simulink model "part2_MAIN_2019_working_EKF"  (R2023a)
settings: Solver=FixedStepAuto  StartTime=0.0  StopTime=500  FixedStep=0.1  RelTol=1e-3
values from neighbouring files (symbols this model uses):
  Af = diag(ti)    [init.m]    (also in init_old.m)
  change_position_time = 400    [init.m]    (also in init_old.m = 1200)
  Gamma = diag(omega_is)    [init.m]    (also in init_old.m)
  Kd = [1660451.40544401; 3920391.80535684; 1605063439.04156]    [init.m]    (also in init_old.m)
  Ki = [137.081306245593; 763.274947400198; 335358.448218978]    [init.m]    (also in init_old.m = [137.081306245593; 3163.274947400198; 335358.448218978])
  Kp = [75459.3345349083; 277551.73586971; 120744473.878042]    [init.m]    (also in init_old.m)
  Omega = diag([omega_n, omega_n, omega_n])    [get_observer_parameters.m]    (also in init.m = diag(2*omega_is.*zeta_is); init_old.m = diag(2*omega_is.*zeta_is))
  simulation = 1    [init.m]    (also in init_old.m)
  vessel =     [test.mat]
undefined symbols (not defined in the file or in its folder): Hoerner, thrusters
libraries: simulink x2, marine_hydro x2, marine_gnc x1
settings Model: PacingRate=8  Creator=jonbjor  LastModifiedBy=goks
settings SolverCC: AlgebraicLoopSolver=TrustRegion
settings DataIOCC: ReturnWorkspaceOutputs=off
settings DebuggingCC: AlgebraicLoopMsg=none  ArtificialAlgebraicLoopMsg=none  UnconnectedInputMsg=warning  UnconnectedOutputMsg=warning  UnconnectedLineMsg=warning  ArithmeticOperatorsInVariantConditions=warning
settings ModelReferenceCC: EnableRefExpFcnMdlSchedulingChecks=on
settings SFSimCC: SimUseLocalCustomCode=off  CustomCodeUndefinedFunction=UseInterfaceOnly
settings RTWCC: RTWUseLocalCustomCode=off  DLArmComputeVersion=19.05

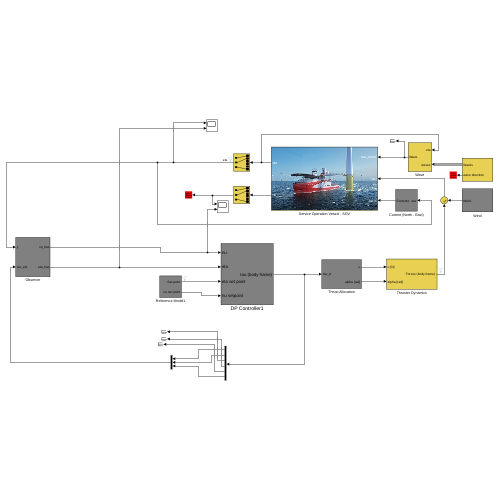
[thumbnail: Simulink's stored preview of the top-level diagram]
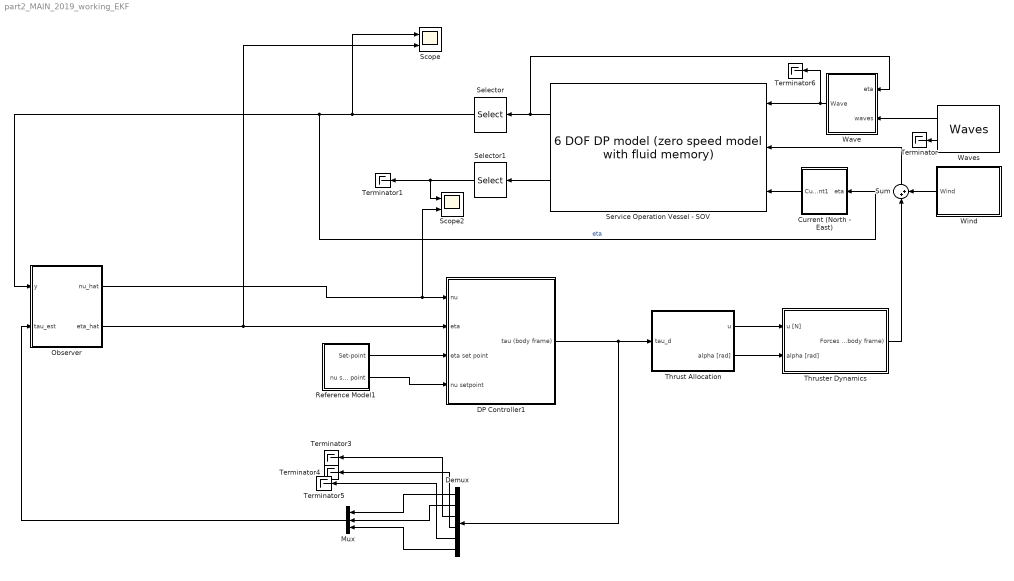
== system part2_MAIN_2019_working_EKF ==
  Current (North - East) : Subsystem
  DP Controller1 : Subsystem
  Demux : Demux  Outputs=6
  Mux : Mux  Inputs=3
  Observer : Subsystem
  Reference Model1 : Subsystem
  Scope : Scope  NumInputPorts=2
  Scope2 : Scope  NumInputPorts=2
  Selector : Selector  InputPortWidth=6  IndexOptions=Index vector (dialog)  Indices=[1 2 6]  OutputSizes=1
  Selector1 : Selector  InputPortWidth=6  IndexOptions=Index vector (dialog)  Indices=[1 2 6]  OutputSizes=1
  Service Operation Vessel - SOV : marine_hydro/Hydro Library/6 DOF DP model  (zero speed model with fluid memory)  ABC=vesselABC  rho=1025  Axc=0.9*vessel.main.T*vessel.main.B  Ayc=0.9*vessel.main.T*vessel.main.Lpp  CX=1  CY_2D=Hoerner(vessel.main.B,vessel.main.T)  Bv=vessel.Bv  mask(6 DOF zero speed model){}
      link override "Integrator1 ": InitialCondition=nu0
      link override Integrator2: InitialCondition=eta0
      mask Display:
      | image('SOV.jpg');
      | color('white'); port_label('output', 1, 'eta')
      | color('white'); port_label('output', 2, 'nu')
      | color('white'); port_label('input', 1, 'tau_wave')
      | color('white'); port_label('input', 2, 'tau')
      | color('white'); port_label('input', 3, 'nu_c')
  Sum : Sum  Inputs=|++
  Terminator{,1,3..6} (6 alike) : Terminator
  Thrust Allocation : Subsystem
  Thruster Dynamics : Subsystem  mask{thrusterfault=off}
      mask prompts: thrusterfault "Fault on thruster #2 and #4?"
  Wave : Subsystem  mask{waveforces=on}
      mask prompts: waveforces "Waveforces enabled"
  Waves : marine_gnc/Environment/Waves/Waves  spectrum_type=ITTC  disp_flag=on  plot_spectrum=off  plot_realization=off  hs=5  omega_peak=pi/10  psi_mean=0  gamma=-1  spread=2  depth=inf  nfreq=20  ndir=10  energylim=0.005  freq_cutoff=3  dir_cutoff=0  rand_seed=123  rand_freq=on  rand_dir=on  Zeta_a=0  Omega=0  Phase=0  Wavenum=0  Psi=0
  Wind : Subsystem
  wires:
  Service Operation Vessel - SOV/2 -> Selector1/1
  Reference Model1/1(Set-point) -> DP Controller1/3(eta set point)
  Service Operation Vessel - SOV/1 -> Wave/1(eta), Selector/1
  Waves/1 -> Wave/2(waves)
  Waves/2 -> Terminator/1
  Sum/1 -> Service Operation Vessel - SOV/2
  Selector/1 -> Scope/1, Current (North - East)/1(eta), Observer/1(y)  "eta"
  Reference Model1/2(nu set point) -> DP Controller1/4(nu setpoint)
  Selector1/1 -> Scope2/1, Terminator1/1
  Current (North - East)/1(Current1) -> Service Operation Vessel - SOV/3
  Wind/1(Wind) -> Sum/2
  Observer/1(nu_hat) -> Scope2/2, DP Controller1/1(nu)
  Demux/1 -> Mux/1
  Demux/2 -> Mux/2
  Demux/6 -> Mux/3
  Mux/1 -> Observer/2(tau_est)
  Demux/3 -> Terminator3/1
  Demux/4 -> Terminator4/1
  Demux/5 -> Terminator5/1
  Wave/1(Wave) -> Service Operation Vessel - SOV/1, Terminator6/1
  Observer/2(eta_hat) -> Scope/2, DP Controller1/2(eta)
  DP Controller1/1(tau (body frame)) -> Thrust Allocation/1(tau_d), Demux/1
  Thrust Allocation/1(u) -> Thruster Dynamics/1(u [N])
  Thruster Dynamics/1("Forces (body frame) ") -> Sum/1
  Thrust Allocation/2(alpha [rad]) -> Thruster Dynamics/2(alpha [rad])

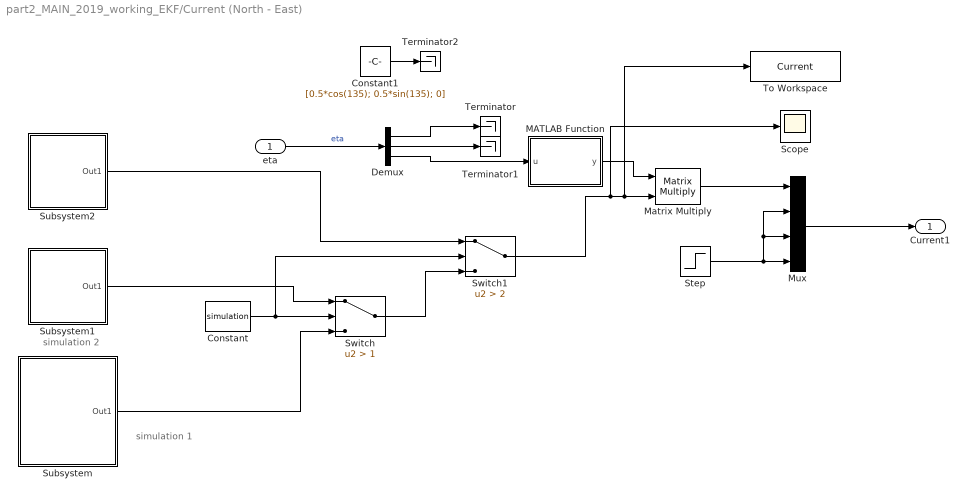
== system part2_MAIN_2019_working_EKF/Current (North - East) ==
  note: simulation 2
  note: simulation 1
  eta : Inport
  Constant : Constant  Value=simulation
  Constant1 : Constant  Value=[0.5*cos(135); 0.5*sin(135); 0]
  Demux : Demux  Outputs=3
  MATLAB Function : MATLAB Function  TreatAsAtomicUnit=on
  Matrix Multiply : Product  Multiplication=Matrix(*)
  Mux : Mux
  Scope : Scope
  Step : Step  After=0  SampleTime=0
  Subsystem : Subsystem
  Subsystem1 : Subsystem
  Subsystem2 : Subsystem
  Switch : Switch  Criteria=u2 > Threshold  Threshold=1  SaturateOnIntegerOverflow=off  InputSameDT=off
  Switch1 : Switch  Criteria=u2 > Threshold  Threshold=2  SaturateOnIntegerOverflow=off  InputSameDT=off
  Terminator : Terminator
  Terminator1 : Terminator
  Terminator2 : Terminator
  To Workspace : ToWorkspace  VariableName=Current  SaveFormat=Timeseries  SampleTime=-1
  Current1 : Outport  VectorParamsAs1DForOutWhenUnconnected=off
  wires:
  Demux/2 -> Terminator1/1
  MATLAB Function/1(y) -> Matrix Multiply/1
  Switch/1 -> Switch1/3
  Matrix Multiply/1 -> Mux/1
  Subsystem2/1(Out1) -> Switch1/1
  Subsystem/1(Out1) -> Switch/3
  Subsystem1/1(Out1) -> Switch/1
  Demux/1 -> Terminator/1
  Switch1/1 -> Scope/1, To Workspace/1, Matrix Multiply/2
  eta/1 -> Demux/1  "eta"
  Constant/1 -> Switch1/2, Switch/2
  Constant1/1 -> Terminator2/1
  Step/1 -> Mux/3, Mux/2, Mux/4
  Demux/3 -> MATLAB Function/1(u)
  Mux/1 -> Current1/1

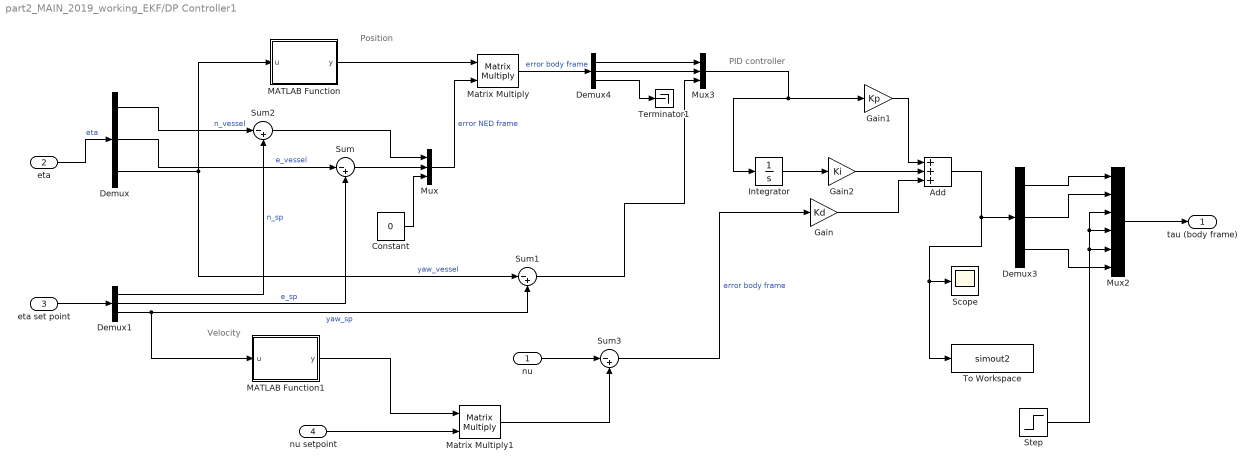
== system part2_MAIN_2019_working_EKF/DP Controller1 ==
  note: PID controller
  note: Velocity
  note: Position
  nu : Inport
  eta : Inport  Port=2
  eta set point : Inport  Port=3
  nu setpoint : Inport  Port=4
  Add : Sum  Inputs=+++
  Constant : Constant  Value=0
  Demux{,1,3..4} (4 alike) : Demux  Outputs=3
  Gain : Gain  Gain=Kd
  Gain1 : Gain  Gain=Kp
  Gain2 : Gain  Gain=Ki
  Integrator : Integrator
  MATLAB Function : MATLAB Function  TreatAsAtomicUnit=on
  MATLAB Function1 : MATLAB Function  TreatAsAtomicUnit=on
  Matrix Multiply : Product  Multiplication=Matrix(*)
  Matrix Multiply1 : Product  Multiplication=Matrix(*)
  Mux : Mux  Inputs=3
  Mux2 : Mux  Inputs=6
  Mux3 : Mux  Inputs=3
  Scope : Scope
  Step : Step  After=0  SampleTime=0
  Sum{,1..3} (4 alike) : Sum  Inputs=|-+
  Terminator1 : Terminator
  To Workspace : ToWorkspace  VariableName=simout2  SaveFormat=Timeseries  SampleTime=-1
  tau (body frame) : Outport  VectorParamsAs1DForOutWhenUnconnected=off
  wires:
  eta/1 -> Demux/1  "eta"
  eta set point/1 -> Demux1/1
  Demux/1 -> Sum2/1  "n_vessel"
  Demux1/1 -> Sum2/2  "n_sp"
  Demux/2 -> Sum/1  "e_vessel"
  Demux1/2 -> Sum/2  "e_sp"
  Sum2/1 -> Mux/1
  Sum/1 -> Mux/2
  MATLAB Function/1(y) -> Matrix Multiply/1
  Mux/1 -> Matrix Multiply/2  "error NED frame"
  Step/1 -> Mux2/4, Mux2/3, Mux2/5
  Demux1/3 -> MATLAB Function1/1(u), Sum1/2  "yaw_sp"
  Sum1/1 -> Mux3/3
  Constant/1 -> Mux/3
  Demux/3 -> Sum1/1, MATLAB Function/1(u)  "yaw_vessel"
  Matrix Multiply/1 -> Demux4/1  "error body frame"
  nu/1 -> Sum3/1
  Sum3/1 -> Gain/1  "error body frame"
  nu setpoint/1 -> Matrix Multiply1/2
  MATLAB Function1/1(y) -> Matrix Multiply1/1
  Matrix Multiply1/1 -> Sum3/2
  Integrator/1 -> Gain2/1
  Gain1/1 -> Add/1
  Gain2/1 -> Add/2
  Gain/1 -> Add/3
  Add/1 -> To Workspace/1, Scope/1, Demux3/1
  Demux3/1 -> Mux2/1
  Demux3/2 -> Mux2/2
  Demux3/3 -> Mux2/6
  Mux2/1 -> tau (body frame)/1
  Demux4/1 -> Mux3/1
  Demux4/2 -> Mux3/2
  Demux4/3 -> Terminator1/1
  Mux3/1 -> Integrator/1, Gain1/1

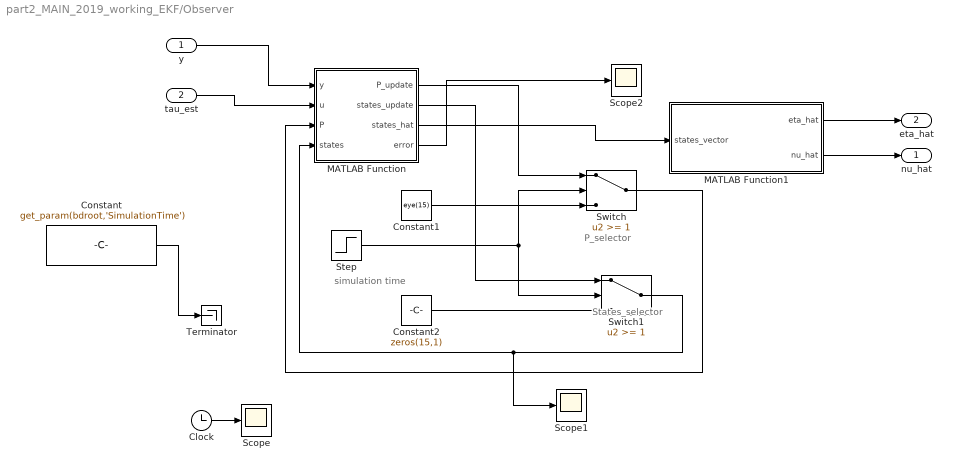
== system part2_MAIN_2019_working_EKF/Observer ==
  note: simulation time
  note: States_selector
  note: P_selector
  y : Inport
  tau_est : Inport  Port=2
  Clock : Clock
  Constant : Constant  Value=get_param(bdroot,'SimulationTime')
  Constant1 : Constant  Value=eye(15)
  Constant2 : Constant  Value=zeros(15,1)
  MATLAB Function : MATLAB Function  TreatAsAtomicUnit=on
  MATLAB Function1 : MATLAB Function  TreatAsAtomicUnit=on
  Scope : Scope
  Scope1 : Scope
  Scope2 : Scope
  Step : Step  Time=0.01  SampleTime=0.1
  Switch : Switch  Threshold=1  SaturateOnIntegerOverflow=off  InputSameDT=off
  Switch1 : Switch  Threshold=1  SaturateOnIntegerOverflow=off  InputSameDT=off
  Terminator : Terminator
  nu_hat : Outport  VectorParamsAs1DForOutWhenUnconnected=off
  eta_hat : Outport  Port=2  VectorParamsAs1DForOutWhenUnconnected=off
  wires:
  tau_est/1 -> MATLAB Function/2(u)
  MATLAB Function/1(P_update) -> Switch/1
  Constant1/1 -> Switch/3
  Constant2/1 -> Switch1/3
  MATLAB Function/2(states_update) -> Switch1/1
  y/1 -> MATLAB Function/1(y)
  Switch/1 -> MATLAB Function/3(P)
  Switch1/1 -> Scope1/1, MATLAB Function/4(states)
  MATLAB Function1/1(eta_hat) -> eta_hat/1
  MATLAB Function1/2(nu_hat) -> nu_hat/1
  Step/1 -> Switch1/2, Switch/2
  Constant/1 -> Terminator/1
  Clock/1 -> Scope/1
  MATLAB Function/3(states_hat) -> MATLAB Function1/1(states_vector)
  MATLAB Function/4(error) -> Scope2/1

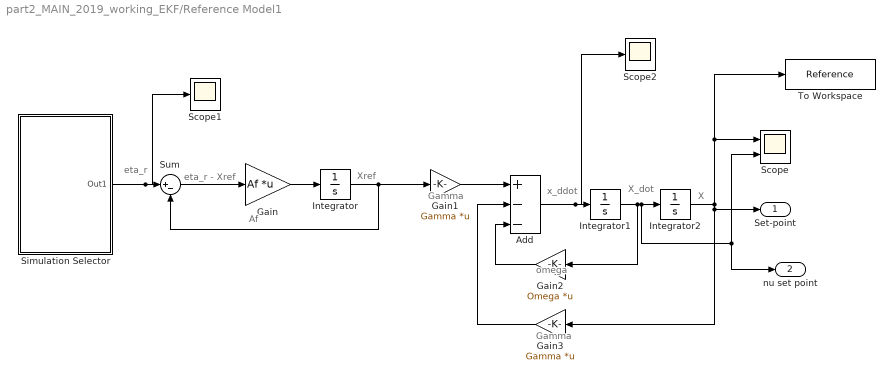
== system part2_MAIN_2019_working_EKF/Reference Model1 ==
  note: Af
  note: eta_r
  note: Xref
  note: omega
  note: eta_r - Xref
  note: Gamma
  note: x_ddot
  note: Gamma
  note: X_dot
  note: X
  Add : Sum  Inputs=+--
  Gain : Gain  Gain=Af  Multiplication=Matrix(K*u)
  Gain1 : Gain  Gain=Gamma  Multiplication=Matrix(K*u)
  Gain2 : Gain  Gain=Omega  Multiplication=Matrix(K*u)
  Gain3 : Gain  Gain=Gamma  Multiplication=Matrix(K*u)
  Integrator : Integrator
  Integrator1 : Integrator
  Integrator2 : Integrator
  Scope : Scope  NumInputPorts=2
  Scope1 : Scope
  Scope2 : Scope
  Simulation Selector : Subsystem
  Sum : Sum  Inputs=|+-
  To Workspace : ToWorkspace  VariableName=Reference  SaveFormat=Timeseries  SampleTime=-1
  Set-point : Outport  VectorParamsAs1DForOutWhenUnconnected=off
  nu set point : Outport  Port=2  VectorParamsAs1DForOutWhenUnconnected=off
  wires:
  Integrator/1 -> Gain1/1, Sum/2
  Add/1 -> Scope2/1, Integrator1/1
  Integrator2/1 -> To Workspace/1, Scope/1, Set-point/1, Gain3/1
  Gain1/1 -> Add/1
  Integrator1/1 -> nu set point/1, Scope/2, Integrator2/1, Gain2/1
  Gain/1 -> Integrator/1
  Gain2/1 -> Add/3
  Gain3/1 -> Add/2
  Simulation Selector/1(Out1) -> Scope1/1, Sum/1
  Sum/1 -> Gain/1

== system part2_MAIN_2019_working_EKF/Thrust Allocation ==
  tau_d : Inport
  MATLAB Function : MATLAB Function  TreatAsAtomicUnit=on
  u : Outport  VectorParamsAs1DForOutWhenUnconnected=off
  alpha [rad] : Outport  Port=2  VectorParamsAs1DForOutWhenUnconnected=off
  wires:
  tau_d/1 -> MATLAB Function/1(tau_d)
  MATLAB Function/1(Td) -> u/1
  MATLAB Function/2(alpha) -> alpha [rad]/1

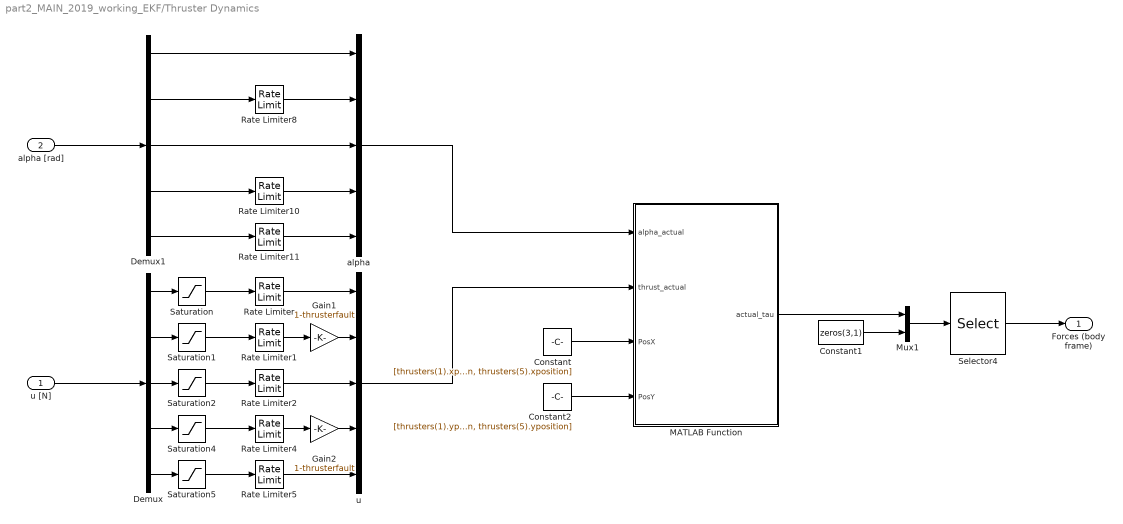
== system part2_MAIN_2019_working_EKF/Thruster Dynamics ==
  u [N] : Inport
  alpha [rad] : Inport  Port=2
  Constant : Constant  Value=[thrusters(1).xposition, thrusters(2).xposition, thrusters(3).xposition, thrusters(4).xposition, thrusters(5).xposition]
  Constant1 : Constant  Value=zeros(3,1)
  Constant2 : Constant  Value=[thrusters(1).yposition, thrusters(2).yposition, thrusters(3).yposition, thrusters(4).yposition, thrusters(5).yposition]
  Demux : Demux  Outputs=5
  Demux1 : Demux  Outputs=5
  Gain1 : Gain  Gain=1-thrusterfault
  Gain2 : Gain  Gain=1-thrusterfault
  MATLAB Function : MATLAB Function  TreatAsAtomicUnit=on
  Mux1 : Mux  Inputs=2
  Rate Limiter : RateLimiter  RisingSlewLimit=thrusters(1).rate  FallingSlewLimit=-thrusters(1).rate  SampleTimeMode=inherited
  Rate Limiter1 : RateLimiter  RisingSlewLimit=thrusters(2).rate  FallingSlewLimit=-thrusters(2).rate  SampleTimeMode=inherited
  Rate Limiter10 : RateLimiter  RisingSlewLimit=thrusters(4).rotationspeed  FallingSlewLimit=-thrusters(4).rotationspeed  SampleTimeMode=inherited
  Rate Limiter11 : RateLimiter  RisingSlewLimit=thrusters(5).rotationspeed  FallingSlewLimit=-thrusters(5).rotationspeed  SampleTimeMode=inherited
  Rate Limiter2 : RateLimiter  RisingSlewLimit=thrusters(3).rate  FallingSlewLimit=-thrusters(3).rate  SampleTimeMode=inherited
  Rate Limiter4 : RateLimiter  RisingSlewLimit=thrusters(4).rate  FallingSlewLimit=-thrusters(4).rate  SampleTimeMode=inherited
  Rate Limiter5 : RateLimiter  RisingSlewLimit=thrusters(5).rate  FallingSlewLimit=-thrusters(5).rate  SampleTimeMode=inherited
  Rate Limiter8 : RateLimiter  RisingSlewLimit=thrusters(2).rotationspeed  FallingSlewLimit=-thrusters(2).rotationspeed  SampleTimeMode=inherited
  Saturation : Saturate  UpperLimit=thrusters(1).thrust  LowerLimit=-thrusters(1).thrust
  Saturation1 : Saturate  UpperLimit=thrusters(2).thrust  LowerLimit=-thrusters(2).thrust
  Saturation2 : Saturate  UpperLimit=thrusters(3).thrust  LowerLimit=-thrusters(3).thrust
  Saturation4 : Saturate  UpperLimit=thrusters(4).thrust  LowerLimit=-thrusters(4).thrust
  Saturation5 : Saturate  UpperLimit=thrusters(5).thrust  LowerLimit=-thrusters(5).thrust
  Selector4 : Selector  InputPortWidth=6  IndexOptions=Index vector (dialog)  Indices=[1 2 4 5 6 3]  OutputSizes=1
  alpha : Mux  Inputs=5
  u : Mux  Inputs=5
  "Forces (body frame) " : Outport  VectorParamsAs1DForOutWhenUnconnected=off
  wires:
  Rate Limiter2/1 -> u/3
  Saturation/1 -> Rate Limiter/1
  Mux1/1 -> Selector4/1
  Constant1/1 -> Mux1/2
  Saturation4/1 -> Rate Limiter4/1
  Demux/2 -> Saturation1/1
  Saturation1/1 -> Rate Limiter1/1
  Demux/1 -> Saturation/1
  Demux/3 -> Saturation2/1
  Saturation2/1 -> Rate Limiter2/1
  Selector4/1 -> "Forces (body frame) "/1
  Gain1/1 -> u/2
  Rate Limiter1/1 -> Gain1/1
  Rate Limiter/1 -> u/1
  Rate Limiter4/1 -> Gain2/1
  Saturation5/1 -> Rate Limiter5/1
  u [N]/1 -> Demux/1
  alpha [rad]/1 -> Demux1/1
  Constant/1 -> MATLAB Function/3(PosX)
  Constant2/1 -> MATLAB Function/4(PosY)
  u/1 -> MATLAB Function/2(thrust_actual)
  alpha/1 -> MATLAB Function/1(alpha_actual)
  MATLAB Function/1(actual_tau) -> Mux1/1
  Rate Limiter10/1 -> alpha/4
  Demux1/4 -> Rate Limiter10/1
  Demux1/5 -> Rate Limiter11/1
  Rate Limiter11/1 -> alpha/5
  Demux1/1 -> alpha/1
  Gain2/1 -> u/4
  Demux/4 -> Saturation4/1
  Demux/5 -> Saturation5/1
  Rate Limiter5/1 -> u/5
  Demux1/2 -> Rate Limiter8/1
  Rate Limiter8/1 -> alpha/2
  Demux1/3 -> alpha/3

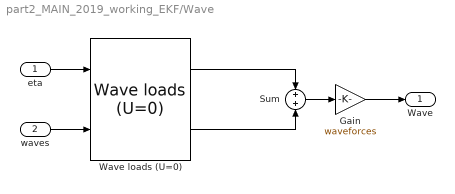
== system part2_MAIN_2019_working_EKF/Wave ==
  eta : Inport
  waves : Inport  Port=2
  Gain : Gain  Gain=waveforces
  Sum : Sum
  Wave loads (U=0) : marine_hydro/Hydro Library/Wave loads (U=0)  SystemSampleTime=-1  VariantActivationTime=update diagram  Latency=0  AutoFrameSizeCalculation=off
  Wave : Outport  VectorParamsAs1DForOutWhenUnconnected=off
  wires:
  eta/1 -> Wave loads (U=0)/1
  waves/1 -> Wave loads (U=0)/2
  Sum/1 -> Gain/1
  Wave loads (U=0)/1 -> Sum/1
  Wave loads (U=0)/2 -> Sum/2
  Gain/1 -> Wave/1

== system part2_MAIN_2019_working_EKF/Wind ==
  Constant : Constant  Value=zeros(6,1)
  Wind : Outport  VectorParamsAs1DForOutWhenUnconnected=off
  wires:
  Constant/1 -> Wind/1

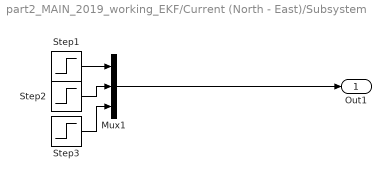
== system part2_MAIN_2019_working_EKF/Current (North - East)/Subsystem ==
  Mux1 : Mux  Inputs=3
  Step1 : Step  Time=0  After=0.5*cos(135)  SampleTime=0
  Step2 : Step  Time=0  After=0.5*sin(135)  SampleTime=0
  Step3 : Step  Time=0  After=0  SampleTime=0
  Out1 : Outport
  wires:
  Mux1/1 -> Out1/1
  Step1/1 -> Mux1/1
  Step2/1 -> Mux1/2
  Step3/1 -> Mux1/3

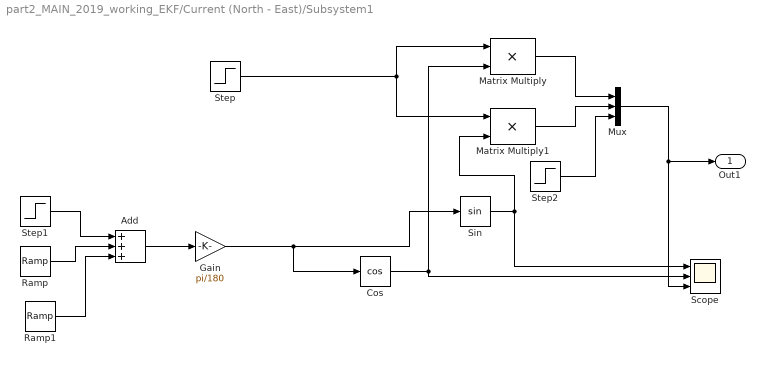
== system part2_MAIN_2019_working_EKF/Current (North - East)/Subsystem1 ==
  Add : Sum  Inputs=+++
  Cos : Trigonometry  Operator=cos
  Gain : Gain  Gain=pi/180
  Matrix Multiply : Product
  Matrix Multiply1 : Product
  Mux : Mux  Inputs=3
  Ramp : simulink/Sources/Ramp  slope=0.45  start=2  InitialOutput=0
  Ramp1 : simulink/Sources/Ramp  slope=-0.45  start=202  InitialOutput=0
  Scope : Scope  NumInputPorts=3
  Sin : Trigonometry
  Step : Step  Time=2  After=0.5  SampleTime=0
  Step1 : Step  Time=2  Before=180  After=180  SampleTime=0
  Step2 : Step  Time=0  After=0  SampleTime=0
  Out1 : Outport
  wires:
  Step1/1 -> Add/1
  Ramp/1 -> Add/2
  Ramp1/1 -> Add/3
  Step/1 -> Matrix Multiply1/1, Matrix Multiply/1
  Sin/1 -> Matrix Multiply1/2, Scope/1
  Cos/1 -> Matrix Multiply/2, Scope/2
  Matrix Multiply/1 -> Mux/1
  Matrix Multiply1/1 -> Mux/2
  Step2/1 -> Mux/3
  Mux/1 -> Scope/3, Out1/1
  Add/1 -> Gain/1
  Gain/1 -> Sin/1, Cos/1

== system part2_MAIN_2019_working_EKF/Current (North - East)/Subsystem2 ==
  Mux : Mux  Inputs=3
  Step : Step  Time=0  After=0  SampleTime=0
  Out1 : Outport
  wires:
  Mux/1 -> Out1/1
  Step/1 -> Mux/3, Mux/2, Mux/1

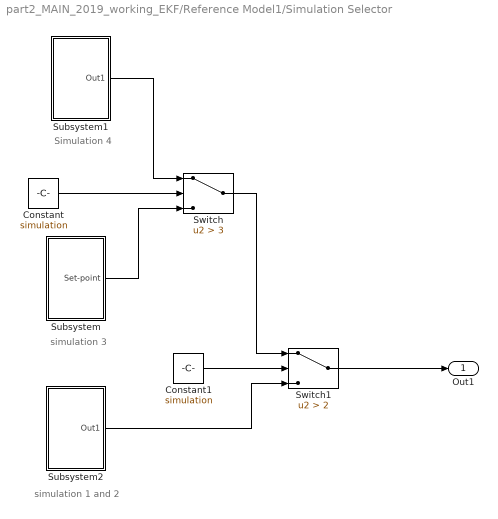
== system part2_MAIN_2019_working_EKF/Reference Model1/Simulation Selector ==
  note: simulation 1 and 2
  note: Simulation 4
  note: simulation 3
  Constant : Constant  Value=simulation
  Constant1 : Constant  Value=simulation
  Subsystem : Subsystem
  Subsystem1 : Subsystem
  Subsystem2 : Subsystem
  Switch : Switch  Criteria=u2 > Threshold  Threshold=3  SaturateOnIntegerOverflow=off  InputSameDT=off
  Switch1 : Switch  Criteria=u2 > Threshold  Threshold=2  SaturateOnIntegerOverflow=off  InputSameDT=off
  Out1 : Outport
  wires:
  Subsystem1/1(Out1) -> Switch/1
  Subsystem/1(Set-point) -> Switch/3
  Constant/1 -> Switch/2
  Switch/1 -> Switch1/1
  Constant1/1 -> Switch1/2
  Subsystem2/1(Out1) -> Switch1/3
  Switch1/1 -> Out1/1

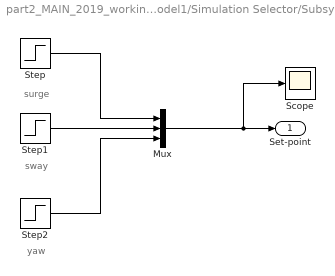
== system part2_MAIN_2019_working_EKF/Reference Model1/Simulation Selector/Subsystem ==
  note: yaw
  note: sway
  note: surge
  Mux : Mux  Inputs=3
  Scope : Scope
  Step : Step  After=10  SampleTime=0
  Step1 : Step  After=10  SampleTime=0
  Step2 : Step  After=3*pi/2  SampleTime=0
  Set-point : Outport
  wires:
  Step/1 -> Mux/1
  Step1/1 -> Mux/2
  Step2/1 -> Mux/3
  Mux/1 -> Scope/1, Set-point/1

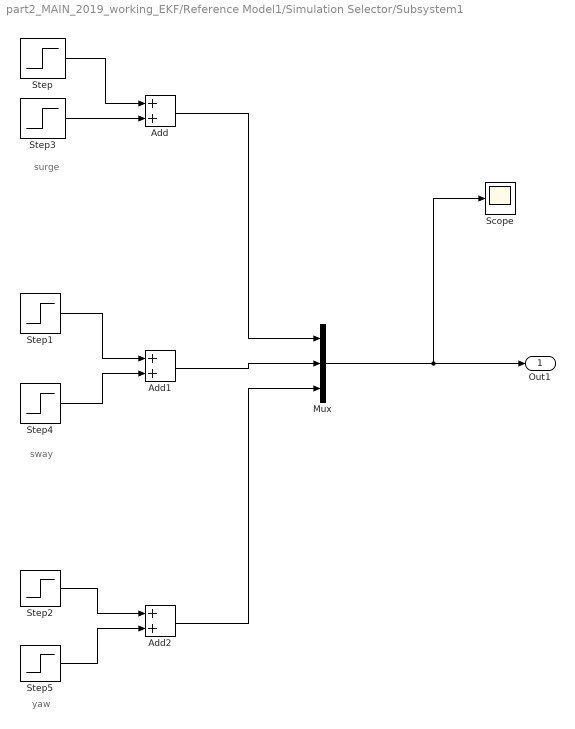
== system part2_MAIN_2019_working_EKF/Reference Model1/Simulation Selector/Subsystem1 ==
  note: yaw
  note: sway
  note: surge
  Add : Sum
  Add1 : Sum
  Add2 : Sum
  Mux : Mux  Inputs=3
  Scope : Scope
  Step : Step  Time=10  After=50  SampleTime=0
  Step1 : Step  Time=change_position_time  After=-50  SampleTime=0
  Step2 : Step  Time=change_position_time*2  After=pi/4  SampleTime=0
  Step3 : Step  Time=change_position_time*3  After=-50  SampleTime=0
  Step4 : Step  Time=change_position_time*4  After=50  SampleTime=0
  Step5 : Step  Time=change_position_time*4  After=-pi/4  SampleTime=0
  Out1 : Outport
  wires:
  Mux/1 -> Scope/1, Out1/1
  Step/1 -> Add/1
  Step3/1 -> Add/2
  Step1/1 -> Add1/1
  Step4/1 -> Add1/2
  Step2/1 -> Add2/1
  Step5/1 -> Add2/2
  Add/1 -> Mux/1
  Add1/1 -> Mux/2
  Add2/1 -> Mux/3

== system part2_MAIN_2019_working_EKF/Reference Model1/Simulation Selector/Subsystem2 ==
  Mux : Mux  Inputs=3
  Step : Step  After=0  SampleTime=0
  Step1 : Step  After=0  SampleTime=0
  Step2 : Step  After=0  SampleTime=0
  Out1 : Outport
  wires:
  Step/1 -> Mux/1
  Step1/1 -> Mux/2
  Step2/1 -> Mux/3
  Mux/1 -> Out1/1

== matlab function part2_MAIN_2019_working_EKF/Current (North - East)/MATLAB Function ==
  data: u input; y output
function y = fcn(u)
rot = [cos(u) -sin(u) 0;
    sin(u) cos(u) 0;
    0 0 1];

y = rot';

== matlab function part2_MAIN_2019_working_EKF/DP Controller1/MATLAB Function ==
  data: u input; y output
function y = fcn(u)

rot = [cos(u) -sin(u) 0;
    sin(u) cos(u) 0;
    0 0 1];

y = rot';

== matlab function part2_MAIN_2019_working_EKF/DP Controller1/MATLAB Function1 ==
  data: u input; y output
function y = fcn(u)

rot = [cos(u) -sin(u) 0;
    sin(u) cos(u) 0;
    0 0 1];

y = rot';

== matlab function part2_MAIN_2019_working_EKF/Observer/MATLAB Function1 ==
  data: states_vector input; eta_hat output; nu_hat output
function [eta_hat, nu_hat] = fcn(states_vector)
%%states [zeta,eta, b, nu] --15x1
%zeta - 6x1, 
%eta - 3x1, 
%b - 3x1, 
%nu - 3x1
eta_hat = states_vector(7:9,1);
nu_hat = states_vector(13:15,1);

end

== matlab function part2_MAIN_2019_working_EKF/Observer/MATLAB Function ==
  data: y input; u input; P input; P_update output; states input; states_update output; states_hat output; error output
function [P_update, states_update,states_hat,error]= fcn(y, u, P, states)
%%%P - 15x15
%states [zeta,eta, b, nu] --15x1
%zeta - 6x1, 
%eta - 3x1, 
%b - 3x1, 
%nu - 3x1
%u - 3x1 force input 
%
%ws_var containing other matrices
%Aw, Tb, B, E, H

%%%all the variables
T_n = 20; %period of interest -- can tune
omega_n = 2* pi / T_n;
zeta = 0.1; %--- can tune
Omega = diag([omega_n, omega_n, omega_n]);
Caret = diag([zeta, zeta, zeta]);
Tb = 0.1 * eye(3); %tune the 0.1
A_w =  [zeros(3) eye(3);
    -Omega^2 -2*Caret*Omega];

ws_var.Aw = A_w;


C_w = [zeros(3) eye(3)];
ws_var.Cw = C_w;



K_w = diag([1, 1, 1]); %-------TUNE
E_w = [zeros(3); K_w];
ws_var.Ew = E_w;
E_b = diag([1, 1, 1]); %-----TUNE 
% Mass = diag([vesselABC.MRB(1,1), vesselABC.MRB(2,2), vesselABC.MRB(6,6)]); %vesselABC.MRB(1:3,1:3);

ws_var.Eb = E_b;
Mass =    [7.0101e+06  0            0;
            0    8.519e+06   4.7187e+05;
            0  4.7187e+05   3.7973e+09];
Damping = diag([2.6486e5, 8.8164e5, 3.3774e8]);
ws_var.M = Mass;
ws_var.D = Damping;

ws_var.B =  [zeros(6,3);zeros(3,3);zeros(3,3);inv(Mass)];
ws_var.E = [E_w, zeros(6,3);
            zeros(3,3), zeros(3,3);
            zeros(3,3), E_b;
            zeros(3,3),zeros(3,3)];
ws_var.H = [C_w, eye(3), zeros(3,3) zeros(3,3)];
ws_var.Tb = Tb;
ws_var.init_state = zeros(15,1);
ws_var.init_Pk = 0.1*eye(15); %tune later
ws_var.R = diag([1,1,0.1]); %tune later
ws_var.Q = diag([1,1,0.1,1e4,1e4,1e5]); %tune this
ws_var.dt = 0.1; %get from simulink fixed step

%%%

H =ws_var.H;
R = ws_var.R;
% y = states(7:9,1);
%predictor
phi = PHI(states,ws_var.dt, ws_var);
TAU = ws_var.dt*ws_var.E;
P_hat = phi*P*phi' + TAU*ws_var.Q*TAU';
states_hat = states+ws_var.dt*F_x_u(states,u, ws_var);


%corrector
%kalman gain
K = P_hat*H'*inv(H*P_hat*H'+R);
P_update = (eye(15)-K*H)*P_hat*(eye(15)-K*H)' + K*R*K';
states_update = states_hat + K*(y-H*states_hat);
error = y - H*states_hat;
end



function phis = PHI(states,dt,ws_var)
%%%states [zeta,eta, b, nu] --15x1
%zeta - 6x1, 
%eta - 3x1, 
%b - 3x1, 
%nu - 3x1
%%%u - 3x1 force input
%%%D - damping, M - Mass, 
%ws_var containing other matrices
%Aw, Tb, B, E, H
zeta = states(1:6,:);
eta = states(7:9,:);
b = states(10:12,:);
nu = states(13:15,:);

psi = eta(3,1);
Jrot = zeros(3,3);
Jrot(1,3) = -cos(psi)*nu(2,1)-sin(psi)*nu(1,1);
Jrot(2,3) = cos(psi)*nu(1,1) - sin(psi)*nu(2,1);

R = [cos(eta(3,1)) -sin(eta(3,1)) 0;
    sin(eta(3,1)) cos(eta(3,1)) 0;
    0 0 1];

phi = zeros(15,15);
phi(1:6,1:6) = ws_var.Aw;
phi(7:9, 7:9) = Jrot;
phi(7:9, 13:15) = R;

phi(10:12, 10:12) = -inv(ws_var.Tb);

phi(13:15, 7:9) = inv(ws_var.M)*[0,0,-sin(eta(3,1))*b(1,1)+b(2,1)*cos(eta(3,1));0,0, -b(1,1)*cos(eta(3,1))-b(2,1)*sin(eta(3,1));0,0,0]; 
phi(13:15,10:12) = inv(ws_var.M)*R' ;%wrt b
phi(13:15, 13:15) = -inv(ws_var.M)*ws_var.D; %wrt nu

phis = eye(15)+dt*phi;
    
end

function Jrot = jac_rot(psi,nu)
Jrot = zeros(3,3);
Jrot(1,3) = -cos(psi)*nu(2,1)-sin(psi)*nu(1,1);
Jrot(2,3) = cos(psi)*nu(1,1) - sin(psi)*nu(2,1);
end
function F = F_x_u(states,u, ws_var)
%%%states [zeta,eta, b, nu] --15x1
%zeta - 6x1, 
%eta - 3x1, 
%b - 3x1, 
%nu - 3x1
%%%u - 3x1 force input
%%%D - damping, M - Mass, 
%ws_var containing other matrices
%Aw, Tb, B, E, H
zeta = states(1:6,:);
eta = states(7:9,:);
b = states(10:12,:);
nu = states(13:15,:);

R = [cos(eta(3,1)) -sin(eta(3,1)) 0;
    sin(eta(3,1)) cos(eta(3,1)) 0;
    0 0 1];

M = ws_var.M;
D = ws_var.D;
Fx = [
ws_var.Aw*zeta;
R*nu;
-inv(ws_var.Tb)*b;
-inv(M)*D*nu + inv(M)*R'*b
];

F = (ws_var.B*u)+Fx;


end

function R = rot(psi)

R = [cos(psi) -sin(psi) 0;
    sin(psi) cos(psi) 0;
    0 0 1];
end

== matlab function part2_MAIN_2019_working_EKF/Thrust Allocation/MATLAB Function ==
  data: tau_d input; Td output; alpha output
function [Td, alpha] = B_redistributed(tau_d)
thr1 = [0 1 39.3].';
thr2_x = [0 1 35.6].';
thr2_y = [1 0 35.6].';
thr3 = [0 1 31.3].';
thr4_x = [0 1 -28.5].';
thr4_y = [1 0 5].';
thr5_x = [0 1 -28.5].';
thr5_y = [1 0 -5].';

B = [thr1 thr2_x thr2_y thr3 thr4_x thr4_y thr5_x thr5_y];

% Expected tau_d dimension : 8x1
tau = [tau_d(1); tau_d(2); tau_d(6)];

Td_r = pinv(B) * tau;

Td = [Td_r(1); 
      sqrt(Td_r(2)^2 + Td_r(3)^2); 
      Td_r(4); 
      sqrt(Td_r(5)^2 + Td_r(6)^2);
      sqrt(Td_r(7)^2 + Td_r(8)^2)];

alpha2 = atan(Td_r(3)/Td_r(2));
alpha4 = atan(Td_r(6)/Td_r(5));
alpha5 = atan(Td_r(8)/Td_r(7));
alpha = [0; alpha2; 0; alpha4; alpha5];

end

== matlab function part2_MAIN_2019_working_EKF/Thruster Dynamics/MATLAB Function ==
  data: alpha_actual input; thrust_actual input; actual_tau output; PosX input; PosY input
function actual_tau   = fcn(alpha_actual,thrust_actual,PosX,PosY)

    Alpha_surge =[cos(alpha_actual(1)) cos(alpha_actual(2)) cos(alpha_actual(3)) cos(alpha_actual(4)) cos(alpha_actual(5))];  
    Alpha_sway = [sin(alpha_actual(1)) sin(alpha_actual(2)) sin(alpha_actual(3)) sin(alpha_actual(4)) sin(alpha_actual(5))];
    Alpha_yaw = [sin(alpha_actual(1))*PosX(1)-cos(alpha_actual(1))*PosY(1) sin(alpha_actual(2))*PosX(2)-cos(alpha_actual(2))*PosY(2) ...
                 sin(alpha_actual(3))*PosX(3)-cos(alpha_actual(3))*PosY(3) sin(alpha_actual(4))*PosX(4)-cos(alpha_actual(4))*PosY(4) ...
                 sin(alpha_actual(5))*PosX(5)-cos(alpha_actual(5))*PosY(5)];

    actual_tau = [Alpha_surge; Alpha_sway; Alpha_yaw]*thrust_actual;
end
